simulink model "purePursuit"  (R2016b)
settings: Solver=VariableStepAuto  StartTime=0.0  StopTime=10.0  RelTol=1e-3
libraries: robotalgslib x1
settings Model: Creator=root  LastModifiedBy=root

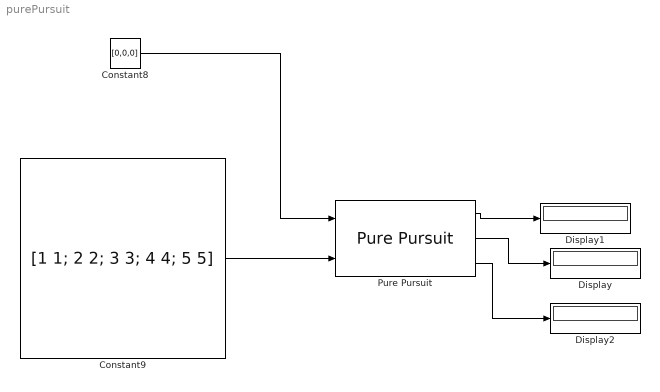
== system purePursuit ==
  Constant8 : Constant  Value=[0,0,0]
  Constant9 : Constant  Value=[1 1; 2 2; 3 3; 4 4; 5 5]
  Display : Display
      settings: Decimation=3
  Display1 : Display
      settings: Decimation=3
  Display2 : Display
      settings: Decimation=3
  Pure Pursuit : robotalgslib/Pure Pursuit  DesiredLinearVelocity=0.1  MaxAngularVelocity=5.0  LookaheadDistance=1.0  TargetDirPort=on  SimulateUsing=Code generation
  wires:
  Pure Pursuit/1 -> Display1/1
  Pure Pursuit/2 -> Display/1
  Constant8/1 -> Pure Pursuit/1
  Constant9/1 -> Pure Pursuit/2
  Pure Pursuit/3 -> Display2/1
